simulink model "DrivetrainHevMm"  (R2021b)
settings: Solver=VariableStepAuto  StartTime=0.0  StopTime=inf  RelTol=1e-3  EnableMultiTasking=on
model workspace (MAT data in the model file):
  DiffRatio : Simulink.Parameter (value not decoded)
  EngDriveRatio : Simulink.Parameter (value not decoded)
  Jengine : Simulink.Parameter (value not decoded)
  MotGbRatio : Simulink.Parameter (value not decoded)
  NF : Simulink.Parameter (value not decoded)
  NR : Simulink.Parameter (value not decoded)
  RWheel : Simulink.Parameter (value not decoded)
  b_axle : Simulink.Parameter (value not decoded)
  b_driveshaft : Simulink.Parameter (value not decoded)
  k_axle : Simulink.Parameter (value not decoded)
  k_driveshaft : Simulink.Parameter (value not decoded)
  wc_shaft : Simulink.Parameter (value not decoded)
symbols that are objects in the model workspace (value not decoded): b_axle, b_driveshaft, EngDriveRatio, k_axle, k_driveshaft, MotGbRatio
libraries: autolibpowerinfoutils x8, autolibsharedcoupling x7, autolibshareddiff x4, autolibshared x3, autolibcoupling x2
(part 3 of 3)

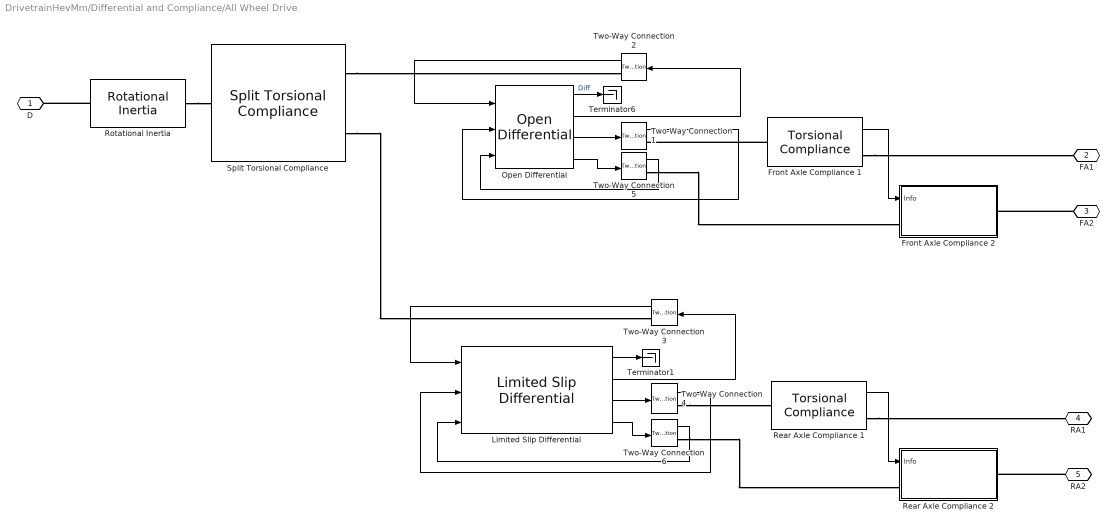
== system DrivetrainHevMm/Differential and Compliance/All Wheel Drive ==
  Front Axle Compliance 1 : autolibsharedcoupling/Torsional Compliance  port_config=Two-way connection  extInfo=on  k=k_axle  b=b_axle  theta_o=0  domega_o=0  omega_c=wc_shaft  blkID=0  aMode=1
      settings: SourceProductBaseCode=PW,DR,MT,UV,VE
  Front Axle Compliance 2 : Subsystem
  Limited Slip Differential : autolibshareddiff/Limited Slip Differential  DiffEffModelPopup=Constant  InterpMethod=Linear point-slope  extTamb=off  shaftSwitchMask=To the left of center-line  Ndiff=DiffRatio  Jd=.025  bd=1e-3  Jw1=.01  bw1=1e-3  Jw2=.01  bw2=1e-3  omegaw1o=0  omegaw2o=0  eta=1  eta_tbl=reshape([0.64 0.76 0.8 0.81 0.83 0.84 0.84 0.56 0.73 0.78 0.8 0.83 0.84 0.84 0.54 0.71 0.77 0.8 0.82 0.84 0.84 0.53 0.71 0.77 0.8 0.83 0.84 0.84 0.51 0.71 0.77 0.8 0.83 0.84 0.85 0.52 0.7 0.77 0.8 0.83 0.84 0.85 0.51 0.71 0.76 0.79 0.83 0.84 0.85 0.5 0.69 0.76 0.79 0.82 0.84 0.85 0.45 0.68 0.75 0.78 0.82 0.84 0.85 0.43 0.67 0.74 0.78 0.81 0.83 0.84 0.38 0.63 0.71 0.75 0.8 0.82 0.83 0.81 0.86 0.88 0.89 0.89 0.89 0.9 0.77 0.85 0.87 0.88 0.89 0.9 0.9 0.72 0.82 0.86 0.87 0.88 0.89 0.9 0.68 0.8 0.84 0.86 0.88 0.89 0.89 0.67 0.8 0.84 0.86 0.88 0.89 0.9 0.67 0.8 0.84 0.86 0.88 0.89 0.9 0.65 0.8 0.84 0.86 0.88 0.89 0.9 0.64 0.79 0.83 0.86 0.88 0.89 0.9 0.63 0.78 0.83 0.86 0.88 0.89 0.9 0.59 0.76 0.82 0.85 0.87 0.89 0.9 0.53 0.73 0.8 0.83 0.86 0.88 0.89], 7, 11, 2)  Trq_bpts=[25, 50, 75, 100, 150, 200, 250]  omega_bpts=[52.4 78.5 105 131 157 183 209 262 314 419 524]  Temp_bpts=[290 358]  Tamb=297.15  couplingType=Pre-loaded ideal clutch  Ndisks=4  Reff=.20  Fc=500  muc=[.16 0.13 0.115 0.11 0.105 0.1025 0.10125]  dw=[0 10 20 40 60 80 100]  Tdw=[-100, -90, -50, -5, 0, 5, 50, 90, 100]  dwT=[-200, -175, -100, - 50, 0, 50, 100, 175, 200]  TTin=[-200 -175 -100 - 50 0 50 100 175 200]  Tin=[-200 -175 -100 - 50 0 50 100 175 200]  tauC=.01  IdealInterpMethod=Linear point-slope  IdealExtrapMethod=Linear  TdwInterpMethod=Linear point-slope  TdwExtrapMethod=Linear  TTinInterpMethod=Linear point-slope  TTinExtrapMethod=Linear  maxAbsSpd=5e3  aMode=1
      settings: SourceProductBaseCode=PW,DR,MT,UV,VE
  Open Differential : autolibshareddiff/Open Differential  DiffEffModelPopup=Constant  InterpMethod=Linear point-slope  extTamb=off  shaftSwitchMask=To the left of center-line  Ndiff=DiffRatio  Jd=.025  bd=1e-3  Jw1=.01  bw1=1e-3  Jw2=.01  bw2=1e-3  omegaw1o=0  omegaw2o=0  eta=1  eta_tbl=reshape([0.64 0.76 0.8 0.81 0.83 0.84 0.84 0.56 0.73 0.78 0.8 0.83 0.84 0.84 0.54 0.71 0.77 0.8 0.82 0.84 0.84 0.53 0.71 0.77 0.8 0.83 0.84 0.84 0.51 0.71 0.77 0.8 0.83 0.84 0.85 0.52 0.7 0.77 0.8 0.83 0.84 0.85 0.51 0.71 0.76 0.79 0.83 0.84 0.85 0.5 0.69 0.76 0.79 0.82 0.84 0.85 0.45 0.68 0.75 0.78 0.82 0.84 0.85 0.43 0.67 0.74 0.78 0.81 0.83 0.84 0.38 0.63 0.71 0.75 0.8 0.82 0.83 0.81 0.86 0.88 0.89 0.89 0.89 0.9 0.77 0.85 0.87 0.88 0.89 0.9 0.9 0.72 0.82 0.86 0.87 0.88 0.89 0.9 0.68 0.8 0.84 0.86 0.88 0.89 0.89 0.67 0.8 0.84 0.86 0.88 0.89 0.9 0.67 0.8 0.84 0.86 0.88 0.89 0.9 0.65 0.8 0.84 0.86 0.88 0.89 0.9 0.64 0.79 0.83 0.86 0.88 0.89 0.9 0.63 0.78 0.83 0.86 0.88 0.89 0.9 0.59 0.76 0.82 0.85 0.87 0.89 0.9 0.53 0.73 0.8 0.83 0.86 0.88 0.89], 7, 11, 2)  Trq_bpts=[25, 50, 75, 100, 150, 200, 250]  omega_bpts=[52.4 78.5 105 131 157 183 209 262 314 419 524]  Temp_bpts=[290 358]  Tamb=297.15  maxAbsSpd=5e3  aMode=1
      settings: SourceProductBaseCode=PW,DR,MT,UV,VE
  Rear Axle Compliance 1 : autolibsharedcoupling/Torsional Compliance  port_config=Two-way connection  extInfo=on  k=k_axle  b=b_axle  theta_o=0  domega_o=0  omega_c=wc_shaft  blkID=0  aMode=1
      settings: SourceProductBaseCode=PW,DR,MT,UV,VE
  Rear Axle Compliance 2 : Subsystem
  Rotational Inertia : autolibsharedcoupling/Rotational Inertia  port_config=Two-way connection  extInfo=off  externJ=off  J=.01  b=.001  omega_o=0  blkID=0  aMode=1
      settings: SourceProductBaseCode=PW,DR,MT,UV,VE
  Split Torsional Compliance : autolibsharedcoupling/Split Torsional Compliance  port_config=Two-way connection  cplrMode=Shaft split  extInfo=off  k1=5e4  b1=1e2  omega1_c=3000  theta1_o=0  domega1_o=0  k2=5e4  b2=1e2  omega2_c=3000  theta2_o=0  domega2_o=0  blkID=0  aMode=1
      settings: SourceProductBaseCode=PW,DR,MT,UV,VE
  Terminator1 : Terminator
  Terminator6 : Terminator
  Two-Way Connection{1..6} (6 alike) : TwoWayConnection
  D : PMIOPort  Side=Left
  FA1 : PMIOPort  Port=2  Side=Right
  FA2 : PMIOPort  Port=3  Side=Right
  RA1 : PMIOPort  Port=4  Side=Right
  RA2 : PMIOPort  Port=5  Side=Right
  wires:
  Two-Way Connection6/1 -> Limited Slip Differential/3
  Limited Slip Differential/4 -> Two-Way Connection6/1
  Rear Axle Compliance 1/1 -> Rear Axle Compliance 2/1(Info)
  Two-Way Connection5/1 -> Open Differential/3
  Open Differential/4 -> Two-Way Connection5/1
  Front Axle Compliance 1/1 -> Front Axle Compliance 2/1(Info)
  Limited Slip Differential/2 -> Two-Way Connection3/1
  Two-Way Connection4/1 -> Limited Slip Differential/2
  Limited Slip Differential/3 -> Two-Way Connection4/1
  Limited Slip Differential/1 -> Terminator1/1
  Two-Way Connection3/1 -> Limited Slip Differential/1
  Open Differential/2 -> Two-Way Connection2/1
  Open Differential/3 -> Two-Way Connection1/1
  Two-Way Connection1/1 -> Open Differential/2
  Two-Way Connection2/1 -> Open Differential/1
  Open Differential/1 -> Terminator6/1  "Diff"
  connections:
  Two-Way Connection6/RConn1 -- Rear Axle Compliance 2/LConn1
  Rear Axle Compliance 1/RConn1 -- RA1/RConn1
  Two-Way Connection4/RConn1 -- Rear Axle Compliance 1/LConn1
  RA2/RConn1 -- Rear Axle Compliance 2/RConn1
  Front Axle Compliance 1/LConn1 -- Two-Way Connection1/RConn1
  Front Axle Compliance 1/RConn1 -- FA1/RConn1
  FA2/RConn1 -- Front Axle Compliance 2/RConn1
  Two-Way Connection5/RConn1 -- Front Axle Compliance 2/LConn1
  Split Torsional Compliance/RConn2 -- Two-Way Connection3/RConn1
  Split Torsional Compliance/RConn1 -- Two-Way Connection2/RConn1
  Rotational Inertia/LConn1 -- D/RConn1
  Rotational Inertia/RConn1 -- Split Torsional Compliance/LConn1

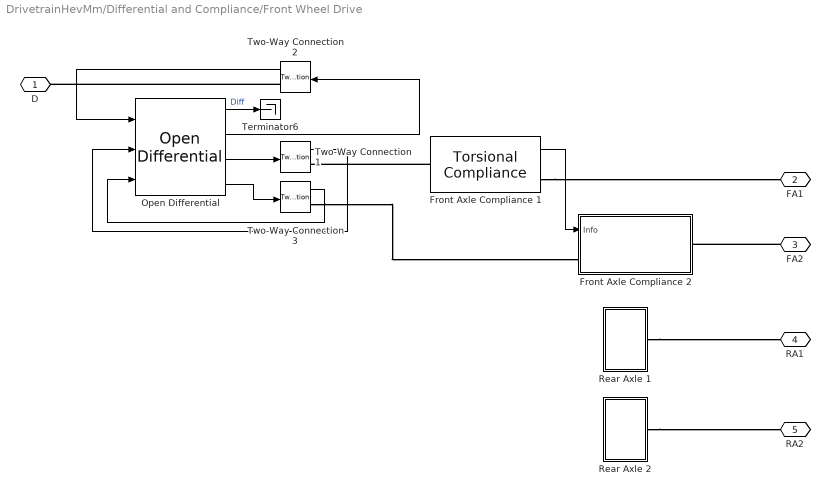
== system DrivetrainHevMm/Differential and Compliance/Front Wheel Drive ==
  Front Axle Compliance 1 : autolibsharedcoupling/Torsional Compliance  port_config=Two-way connection  extInfo=on  k=k_axle  b=b_axle  theta_o=0  domega_o=0  omega_c=wc_shaft  blkID=0  aMode=1
      settings: SourceProductBaseCode=PW,DR,MT,UV,VE
  Front Axle Compliance 2 : Subsystem
  Open Differential : autolibshareddiff/Open Differential  DiffEffModelPopup=Constant  InterpMethod=Linear point-slope  extTamb=off  shaftSwitchMask=To the left of center-line  Ndiff=DiffRatio  Jd=.025  bd=1e-3  Jw1=.01  bw1=1e-3  Jw2=.01  bw2=1e-3  omegaw1o=0  omegaw2o=0  eta=0.97  eta_tbl=reshape([0.64 0.76 0.8 0.81 0.83 0.84 0.84 0.56 0.73 0.78 0.8 0.83 0.84 0.84 0.54 0.71 0.77 0.8 0.82 0.84 0.84 0.53 0.71 0.77 0.8 0.83 0.84 0.84 0.51 0.71 0.77 0.8 0.83 0.84 0.85 0.52 0.7 0.77 0.8 0.83 0.84 0.85 0.51 0.71 0.76 0.79 0.83 0.84 0.85 0.5 0.69 0.76 0.79 0.82 0.84 0.85 0.45 0.68 0.75 0.78 0.82 0.84 0.85 0.43 0.67 0.74 0.78 0.81 0.83 0.84 0.38 0.63 0.71 0.75 0.8 0.82 0.83 0.81 0.86 0.88 0.89 0.89 0.89 0.9 0.77 0.85 0.87 0.88 0.89 0.9 0.9 0.72 0.82 0.86 0.87 0.88 0.89 0.9 0.68 0.8 0.84 0.86 0.88 0.89 0.89 0.67 0.8 0.84 0.86 0.88 0.89 0.9 0.67 0.8 0.84 0.86 0.88 0.89 0.9 0.65 0.8 0.84 0.86 0.88 0.89 0.9 0.64 0.79 0.83 0.86 0.88 0.89 0.9 0.63 0.78 0.83 0.86 0.88 0.89 0.9 0.59 0.76 0.82 0.85 0.87 0.89 0.9 0.53 0.73 0.8 0.83 0.86 0.88 0.89], 7, 11, 2)  Trq_bpts=[25, 50, 75, 100, 150, 200, 250]  omega_bpts=[52.4 78.5 105 131 157 183 209 262 314 419 524]  Temp_bpts=[290 358]  Tamb=297.15  maxAbsSpd=5e3  aMode=1
      settings: SourceProductBaseCode=PW,DR,MT,UV,VE
  Rear Axle 1 : Subsystem
  Rear Axle 2 : Subsystem
  Terminator6 : Terminator
  Two-Way Connection1 : TwoWayConnection
  Two-Way Connection2 : TwoWayConnection
  Two-Way Connection3 : TwoWayConnection
  D : PMIOPort  Side=Left
  FA1 : PMIOPort  Port=2  Side=Right
  FA2 : PMIOPort  Port=3  Side=Right
  RA1 : PMIOPort  Port=4  Side=Right
  RA2 : PMIOPort  Port=5  Side=Right
  wires:
  Two-Way Connection3/1 -> Open Differential/3
  Open Differential/4 -> Two-Way Connection3/1
  Front Axle Compliance 1/1 -> Front Axle Compliance 2/1(Info)
  Open Differential/2 -> Two-Way Connection2/1
  Open Differential/3 -> Two-Way Connection1/1
  Two-Way Connection1/1 -> Open Differential/2
  Two-Way Connection2/1 -> Open Differential/1
  Open Differential/1 -> Terminator6/1  "Diff"
  connections:
  Rear Axle 2/RConn1 -- RA2/RConn1
  Rear Axle 1/RConn1 -- RA1/RConn1
  FA2/RConn1 -- Front Axle Compliance 2/RConn1
  Two-Way Connection3/RConn1 -- Front Axle Compliance 2/LConn1
  Two-Way Connection2/RConn1 -- D/RConn1
  Front Axle Compliance 1/LConn1 -- Two-Way Connection1/RConn1
  Front Axle Compliance 1/RConn1 -- FA1/RConn1

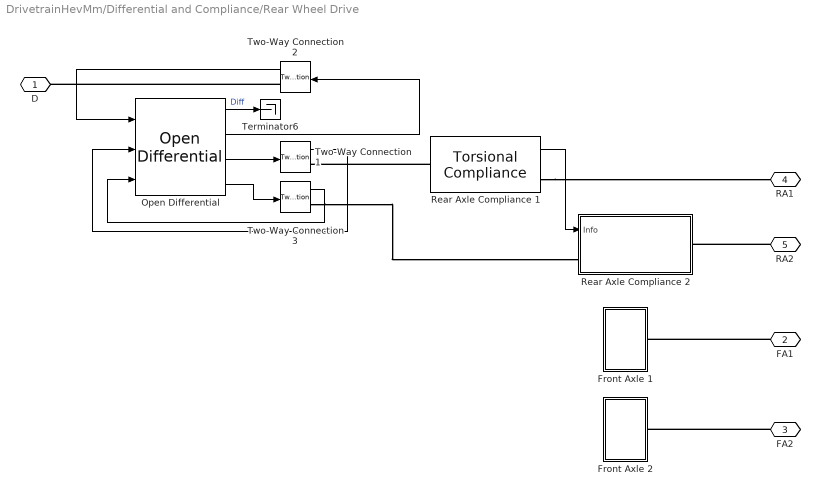
== system DrivetrainHevMm/Differential and Compliance/Rear Wheel Drive ==
  Front Axle 1 : Subsystem
  Front Axle 2 : Subsystem
  Open Differential : autolibshareddiff/Open Differential  DiffEffModelPopup=Constant  InterpMethod=Linear point-slope  extTamb=off  shaftSwitchMask=To the left of center-line  Ndiff=DiffRatio  Jd=.025  bd=1e-3  Jw1=.01  bw1=1e-3  Jw2=.01  bw2=1e-3  omegaw1o=0  omegaw2o=0  eta=1  eta_tbl=reshape([0.64 0.76 0.8 0.81 0.83 0.84 0.84 0.56 0.73 0.78 0.8 0.83 0.84 0.84 0.54 0.71 0.77 0.8 0.82 0.84 0.84 0.53 0.71 0.77 0.8 0.83 0.84 0.84 0.51 0.71 0.77 0.8 0.83 0.84 0.85 0.52 0.7 0.77 0.8 0.83 0.84 0.85 0.51 0.71 0.76 0.79 0.83 0.84 0.85 0.5 0.69 0.76 0.79 0.82 0.84 0.85 0.45 0.68 0.75 0.78 0.82 0.84 0.85 0.43 0.67 0.74 0.78 0.81 0.83 0.84 0.38 0.63 0.71 0.75 0.8 0.82 0.83 0.81 0.86 0.88 0.89 0.89 0.89 0.9 0.77 0.85 0.87 0.88 0.89 0.9 0.9 0.72 0.82 0.86 0.87 0.88 0.89 0.9 0.68 0.8 0.84 0.86 0.88 0.89 0.89 0.67 0.8 0.84 0.86 0.88 0.89 0.9 0.67 0.8 0.84 0.86 0.88 0.89 0.9 0.65 0.8 0.84 0.86 0.88 0.89 0.9 0.64 0.79 0.83 0.86 0.88 0.89 0.9 0.63 0.78 0.83 0.86 0.88 0.89 0.9 0.59 0.76 0.82 0.85 0.87 0.89 0.9 0.53 0.73 0.8 0.83 0.86 0.88 0.89], 7, 11, 2)  Trq_bpts=[25, 50, 75, 100, 150, 200, 250]  omega_bpts=[52.4 78.5 105 131 157 183 209 262 314 419 524]  Temp_bpts=[290 358]  Tamb=297.15  maxAbsSpd=5e3  aMode=1
      settings: SourceProductBaseCode=PW,DR,MT,UV,VE
  Rear Axle Compliance 1 : autolibsharedcoupling/Torsional Compliance  port_config=Two-way connection  extInfo=on  k=k_axle  b=b_axle  theta_o=0  domega_o=0  omega_c=wc_shaft  blkID=0  aMode=1
      settings: SourceProductBaseCode=PW,DR,MT,UV,VE
  Rear Axle Compliance 2 : Subsystem
  Terminator6 : Terminator
  Two-Way Connection1 : TwoWayConnection
  Two-Way Connection2 : TwoWayConnection
  Two-Way Connection3 : TwoWayConnection
  D : PMIOPort  Side=Left
  FA1 : PMIOPort  Port=2  Side=Right
  FA2 : PMIOPort  Port=3  Side=Right
  RA1 : PMIOPort  Port=4  Side=Right
  RA2 : PMIOPort  Port=5  Side=Right
  wires:
  Rear Axle Compliance 1/1 -> Rear Axle Compliance 2/1(Info)
  Open Differential/3 -> Two-Way Connection1/1
  Open Differential/1 -> Terminator6/1  "Diff"
  Two-Way Connection2/1 -> Open Differential/1
  Two-Way Connection1/1 -> Open Differential/2
  Open Differential/2 -> Two-Way Connection2/1
  Open Differential/4 -> Two-Way Connection3/1
  Two-Way Connection3/1 -> Open Differential/3
  connections:
  FA2/RConn1 -- Front Axle 2/RConn1
  FA1/RConn1 -- Front Axle 1/RConn1
  RA2/RConn1 -- Rear Axle Compliance 2/RConn1
  Rear Axle Compliance 1/RConn1 -- RA1/RConn1
  Two-Way Connection2/RConn1 -- D/RConn1
  Two-Way Connection3/RConn1 -- Rear Axle Compliance 2/LConn1
  Rear Axle Compliance 1/LConn1 -- Two-Way Connection1/RConn1

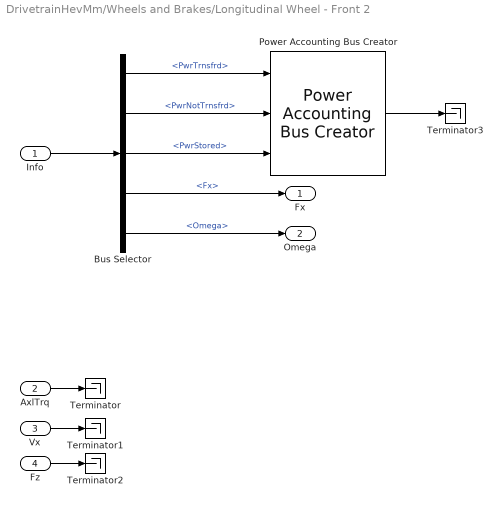
== system DrivetrainHevMm/Wheels and Brakes/Longitudinal Wheel - Front 2 ==
  Info : Inport
  AxlTrq : Inport  Port=2
  Vx : Inport  Port=3
  Fz : Inport  Port=4
  Bus Selector : BusSelector  OutputSignals=PwrInfo.PwrTrnsfrd,PwrInfo.PwrNotTrnsfrd,PwrInfo.PwrStored,Fx,Omega
  Power Accounting Bus Creator : autolibpowerinfoutils/Power Accounting Bus Creator  AssctBlkSelPopup=Parent  RefBlkName='libraryname/blkname'  PwrTrnsfrdCheckBox=on  PwrNotTrnsfrdCheckBox=on  PwrStoredCheckBox=on  aMode=aMode
      settings: SourceProductBaseCode=PW,DR,MT,UV,VE
  Terminator{,1..3} (4 alike) : Terminator
  Fx : Outport  VectorParamsAs1DForOutWhenUnconnected=off
  Omega : Outport  Port=2  VectorParamsAs1DForOutWhenUnconnected=off
  wires:
  Power Accounting Bus Creator/1 -> Terminator3/1
  Bus Selector/5 -> Omega/1  "<Omega>"
  Bus Selector/4 -> Fx/1  "<Fx>"
  Bus Selector/3 -> Power Accounting Bus Creator/3  "<PwrStored>"
  Bus Selector/2 -> Power Accounting Bus Creator/2  "<PwrNotTrnsfrd>"
  Bus Selector/1 -> Power Accounting Bus Creator/1  "<PwrTrnsfrd>"
  Info/1 -> Bus Selector/1
  Fz/1 -> Terminator2/1
  Vx/1 -> Terminator1/1
  AxlTrq/1 -> Terminator/1

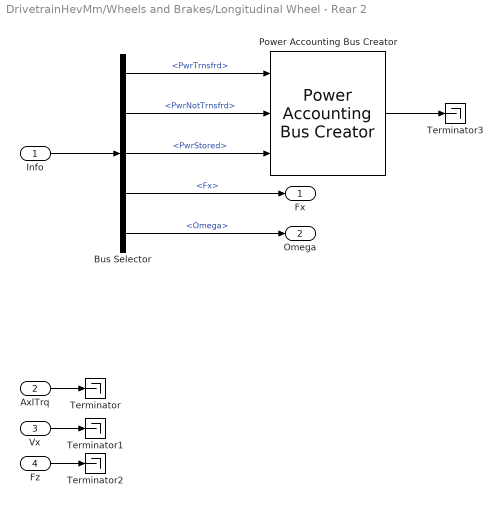
== system DrivetrainHevMm/Wheels and Brakes/Longitudinal Wheel - Rear 2 ==
  Info : Inport
  AxlTrq : Inport  Port=2
  Vx : Inport  Port=3
  Fz : Inport  Port=4
  Bus Selector : BusSelector  OutputSignals=PwrInfo.PwrTrnsfrd,PwrInfo.PwrNotTrnsfrd,PwrInfo.PwrStored,Fx,Omega
  Power Accounting Bus Creator : autolibpowerinfoutils/Power Accounting Bus Creator  AssctBlkSelPopup=Parent  RefBlkName='libraryname/blkname'  PwrTrnsfrdCheckBox=on  PwrNotTrnsfrdCheckBox=on  PwrStoredCheckBox=on  aMode=aMode
      settings: SourceProductBaseCode=PW,DR,MT,UV,VE
  Terminator{,1..3} (4 alike) : Terminator
  Fx : Outport  VectorParamsAs1DForOutWhenUnconnected=off
  Omega : Outport  Port=2  VectorParamsAs1DForOutWhenUnconnected=off
  wires:
  Power Accounting Bus Creator/1 -> Terminator3/1
  Bus Selector/5 -> Omega/1  "<Omega>"
  Bus Selector/4 -> Fx/1  "<Fx>"
  Bus Selector/3 -> Power Accounting Bus Creator/3  "<PwrStored>"
  Bus Selector/2 -> Power Accounting Bus Creator/2  "<PwrNotTrnsfrd>"
  Bus Selector/1 -> Power Accounting Bus Creator/1  "<PwrTrnsfrd>"
  Info/1 -> Bus Selector/1
  Fz/1 -> Terminator2/1
  Vx/1 -> Terminator1/1
  AxlTrq/1 -> Terminator/1

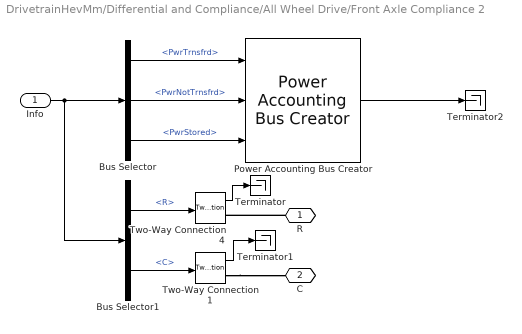
== system DrivetrainHevMm/Differential and Compliance/All Wheel Drive/Front Axle Compliance 2 ==
  Info : Inport
  Bus Selector : BusSelector  OutputSignals=PwrInfo.PwrTrnsfrd,PwrInfo.PwrNotTrnsfrd,PwrInfo.PwrStored
  Bus Selector1 : BusSelector  OutputSignals=Trq.R,Trq.C
  Power Accounting Bus Creator : autolibpowerinfoutils/Power Accounting Bus Creator  AssctBlkSelPopup=Parent  RefBlkName='libraryname/blkname'  PwrTrnsfrdCheckBox=on  PwrNotTrnsfrdCheckBox=on  PwrStoredCheckBox=on  aMode=aMode
      settings: SourceProductBaseCode=PW,DR,MT,UV,VE
  Terminator : Terminator
  Terminator1 : Terminator
  Terminator2 : Terminator
  Two-Way Connection1 : TwoWayConnection
  Two-Way Connection4 : TwoWayConnection
  R : PMIOPort  Side=Left
  C : PMIOPort  Port=2  Side=Right
  wires:
  Bus Selector/3 -> Power Accounting Bus Creator/3  "<PwrStored>"
  Bus Selector/2 -> Power Accounting Bus Creator/2  "<PwrNotTrnsfrd>"
  Bus Selector/1 -> Power Accounting Bus Creator/1  "<PwrTrnsfrd>"
  Power Accounting Bus Creator/1 -> Terminator2/1
  Bus Selector1/2 -> Two-Way Connection1/1  "<C>"
  Bus Selector1/1 -> Two-Way Connection4/1  "<R>"
  Two-Way Connection1/1 -> Terminator1/1
  Info/1 -> Bus Selector/1, Bus Selector1/1
  Two-Way Connection4/1 -> Terminator/1
  connections:
  Two-Way Connection1/RConn1 -- C/RConn1
  R/RConn1 -- Two-Way Connection4/RConn1

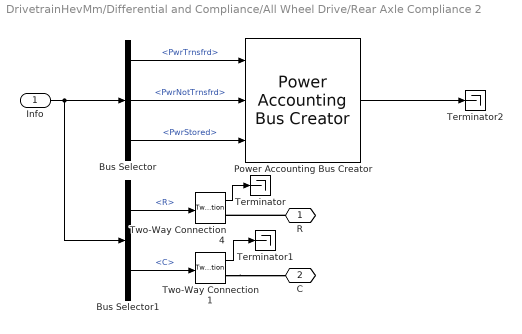
== system DrivetrainHevMm/Differential and Compliance/All Wheel Drive/Rear Axle Compliance 2 ==
  Info : Inport
  Bus Selector : BusSelector  OutputSignals=PwrInfo.PwrTrnsfrd,PwrInfo.PwrNotTrnsfrd,PwrInfo.PwrStored
  Bus Selector1 : BusSelector  OutputSignals=Trq.R,Trq.C
  Power Accounting Bus Creator : autolibpowerinfoutils/Power Accounting Bus Creator  AssctBlkSelPopup=Parent  RefBlkName='libraryname/blkname'  PwrTrnsfrdCheckBox=on  PwrNotTrnsfrdCheckBox=on  PwrStoredCheckBox=on  aMode=aMode
      settings: SourceProductBaseCode=PW,DR,MT,UV,VE
  Terminator : Terminator
  Terminator1 : Terminator
  Terminator2 : Terminator
  Two-Way Connection1 : TwoWayConnection
  Two-Way Connection4 : TwoWayConnection
  R : PMIOPort  Side=Left
  C : PMIOPort  Port=2  Side=Right
  wires:
  Bus Selector/3 -> Power Accounting Bus Creator/3  "<PwrStored>"
  Bus Selector/2 -> Power Accounting Bus Creator/2  "<PwrNotTrnsfrd>"
  Bus Selector/1 -> Power Accounting Bus Creator/1  "<PwrTrnsfrd>"
  Power Accounting Bus Creator/1 -> Terminator2/1
  Bus Selector1/2 -> Two-Way Connection1/1  "<C>"
  Bus Selector1/1 -> Two-Way Connection4/1  "<R>"
  Two-Way Connection1/1 -> Terminator1/1
  Info/1 -> Bus Selector/1, Bus Selector1/1
  Two-Way Connection4/1 -> Terminator/1
  connections:
  Two-Way Connection1/RConn1 -- C/RConn1
  R/RConn1 -- Two-Way Connection4/RConn1

== system DrivetrainHevMm/Differential and Compliance/Front Wheel Drive/Front Axle Compliance 2 ==
  Info : Inport
  Bus Selector : BusSelector  OutputSignals=PwrInfo.PwrTrnsfrd,PwrInfo.PwrNotTrnsfrd,PwrInfo.PwrStored
  Bus Selector1 : BusSelector  OutputSignals=Trq.R,Trq.C
  Power Accounting Bus Creator : autolibpowerinfoutils/Power Accounting Bus Creator  AssctBlkSelPopup=Parent  RefBlkName='libraryname/blkname'  PwrTrnsfrdCheckBox=on  PwrNotTrnsfrdCheckBox=on  PwrStoredCheckBox=on  aMode=aMode
      settings: SourceProductBaseCode=PW,DR,MT,UV,VE
  Terminator : Terminator
  Terminator1 : Terminator
  Terminator2 : Terminator
  Two-Way Connection1 : TwoWayConnection
  Two-Way Connection4 : TwoWayConnection
  R : PMIOPort  Side=Left
  C : PMIOPort  Port=2  Side=Right
  wires:
  Bus Selector/3 -> Power Accounting Bus Creator/3  "<PwrStored>"
  Bus Selector/2 -> Power Accounting Bus Creator/2  "<PwrNotTrnsfrd>"
  Bus Selector/1 -> Power Accounting Bus Creator/1  "<PwrTrnsfrd>"
  Power Accounting Bus Creator/1 -> Terminator2/1
  Bus Selector1/2 -> Two-Way Connection1/1  "<C>"
  Bus Selector1/1 -> Two-Way Connection4/1  "<R>"
  Two-Way Connection1/1 -> Terminator1/1
  Info/1 -> Bus Selector/1, Bus Selector1/1
  Two-Way Connection4/1 -> Terminator/1
  connections:
  Two-Way Connection1/RConn1 -- C/RConn1
  R/RConn1 -- Two-Way Connection4/RConn1

== system DrivetrainHevMm/Differential and Compliance/Front Wheel Drive/Rear Axle 1 ==
  Ground : Ground
  Terminator1 : Terminator
  Two-Way Connection : TwoWayConnection
  RA1 : PMIOPort  Side=Right
  wires:
  Ground/1 -> Two-Way Connection/1
  Two-Way Connection/1 -> Terminator1/1
  connections:
  Two-Way Connection/RConn1 -- RA1/RConn1

== system DrivetrainHevMm/Differential and Compliance/Front Wheel Drive/Rear Axle 2 ==
  Ground1 : Ground
  Terminator : Terminator
  Two-Way Connection4 : TwoWayConnection
  RA2 : PMIOPort  Side=Right
  wires:
  Ground1/1 -> Two-Way Connection4/1
  Two-Way Connection4/1 -> Terminator/1
  connections:
  Two-Way Connection4/RConn1 -- RA2/RConn1

== system DrivetrainHevMm/Differential and Compliance/Rear Wheel Drive/Front Axle 1 ==
  Ground : Ground
  Terminator1 : Terminator
  Two-Way Connection : TwoWayConnection
  FA1 : PMIOPort  Side=Right
  wires:
  Ground/1 -> Two-Way Connection/1
  Two-Way Connection/1 -> Terminator1/1
  connections:
  Two-Way Connection/RConn1 -- FA1/RConn1

== system DrivetrainHevMm/Differential and Compliance/Rear Wheel Drive/Front Axle 2 ==
  Ground1 : Ground
  Terminator : Terminator
  Two-Way Connection4 : TwoWayConnection
  FA2 : PMIOPort  Side=Right
  wires:
  Ground1/1 -> Two-Way Connection4/1
  Two-Way Connection4/1 -> Terminator/1
  connections:
  Two-Way Connection4/RConn1 -- FA2/RConn1

== system DrivetrainHevMm/Differential and Compliance/Rear Wheel Drive/Rear Axle Compliance 2 ==
  Info : Inport
  Bus Selector : BusSelector  OutputSignals=PwrInfo.PwrTrnsfrd,PwrInfo.PwrNotTrnsfrd,PwrInfo.PwrStored
  Bus Selector1 : BusSelector  OutputSignals=Trq.R,Trq.C
  Power Accounting Bus Creator : autolibpowerinfoutils/Power Accounting Bus Creator  AssctBlkSelPopup=Parent  RefBlkName='libraryname/blkname'  PwrTrnsfrdCheckBox=on  PwrNotTrnsfrdCheckBox=on  PwrStoredCheckBox=on  aMode=aMode
      settings: SourceProductBaseCode=PW,DR,MT,UV,VE
  Terminator : Terminator
  Terminator1 : Terminator
  Terminator2 : Terminator
  Two-Way Connection1 : TwoWayConnection
  Two-Way Connection4 : TwoWayConnection
  R : PMIOPort  Side=Left
  C : PMIOPort  Port=2  Side=Right
  wires:
  Bus Selector/3 -> Power Accounting Bus Creator/3  "<PwrStored>"
  Bus Selector/2 -> Power Accounting Bus Creator/2  "<PwrNotTrnsfrd>"
  Bus Selector/1 -> Power Accounting Bus Creator/1  "<PwrTrnsfrd>"
  Power Accounting Bus Creator/1 -> Terminator2/1
  Bus Selector1/2 -> Two-Way Connection1/1  "<C>"
  Bus Selector1/1 -> Two-Way Connection4/1  "<R>"
  Two-Way Connection1/1 -> Terminator1/1
  Info/1 -> Bus Selector/1, Bus Selector1/1
  Two-Way Connection4/1 -> Terminator/1
  connections:
  Two-Way Connection1/RConn1 -- C/RConn1
  R/RConn1 -- Two-Way Connection4/RConn1
